simulink model "exp5"  (R2025b)
settings: Solver=VariableStepAuto  StartTime=0.0  StopTime=10.0  RelTol=1e-3
settings Model: Creator=SUBHASH  LastModifiedBy=SUBHASH

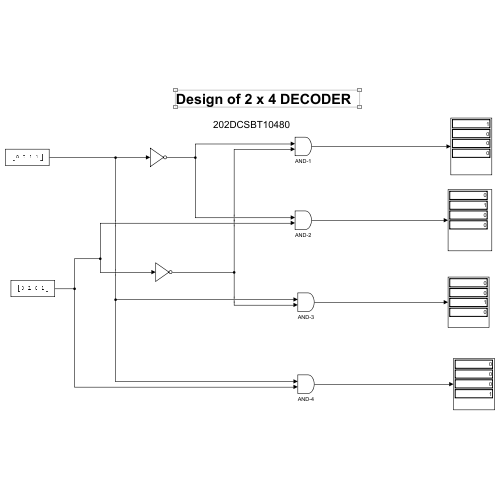
[thumbnail: Simulink's stored preview of the top-level diagram]
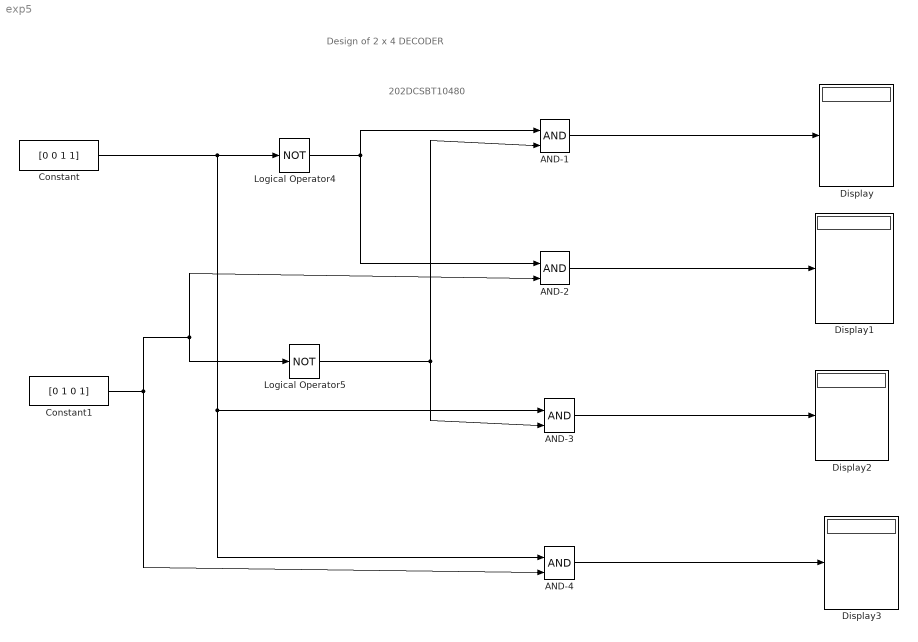
== system exp5 ==
  note: 202DCSBT10480
  note: Design of 2 x 4 DECODER
  AND-{1..4} (4 alike) : Logic  IconShape=distinctive  AllPortsSameDT=off  OutDataTypeStr=boolean
  Constant : Constant  Value=[0 0 1 1]
  Constant1 : Constant  Value=[0 1 0 1]
  Display{,1..3} (4 alike) : Display
      settings: Decimation=4
  Logical Operator4 : Logic  Operator=NOT  IconShape=distinctive  AllPortsSameDT=off  OutDataTypeStr=boolean
  Logical Operator5 : Logic  Operator=NOT  IconShape=distinctive  AllPortsSameDT=off  OutDataTypeStr=boolean
  wires:
  Constant/1 -> Logical Operator4/1, AND-3/1, AND-4/1
  Logical Operator4/1 -> AND-1/1, AND-2/1
  AND-1/1 -> Display/1
  Logical Operator5/1 -> AND-1/2, AND-3/2
  Constant1/1 -> AND-2/2, Logical Operator5/1, AND-4/2
  AND-2/1 -> Display1/1
  AND-3/1 -> Display2/1
  AND-4/1 -> Display3/1
